simulink model "Esercizio7_sim"  (R2022a)
settings: Solver=VariableStepAuto  StartTime=0.0  StopTime=10  RelTol=1e-3
values from neighbouring files (symbols this model uses):
  C_d = c2d(C, Tc, 'tustin')    [Esercizio7.m]    (also in myESE6.m)
  G = tf(num, den)    [Esercizio7.m]    (also in myESE6.m = tf(num,den))
  Tc = 2*pi/ 500    (= 0.0125663706144)    [Esercizio7.m]    (also in SPIEGAZIONE.m = 2*PI/wc; myESE6.m)
settings Model: Creator=chiar  LastModifiedBy=Stefano
settings SolverCC: AlgebraicLoopSolver=TrustRegion
settings DebuggingCC: UnconnectedInputMsg=warning  UnconnectedOutputMsg=warning  UnconnectedLineMsg=warning  SFMachineParentedDataDiag=warning
settings RTWCC: DLArmComputeVersion=19.05

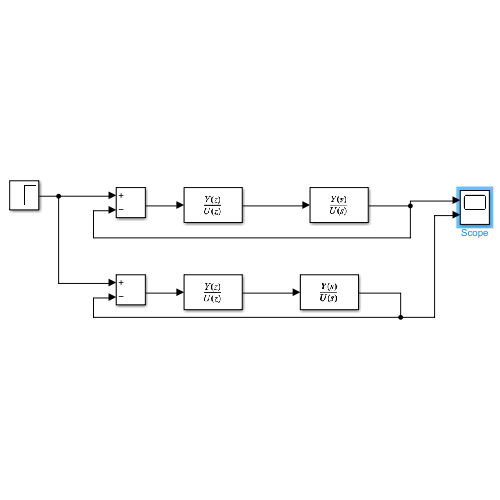
[thumbnail: Simulink's stored preview of the top-level diagram]
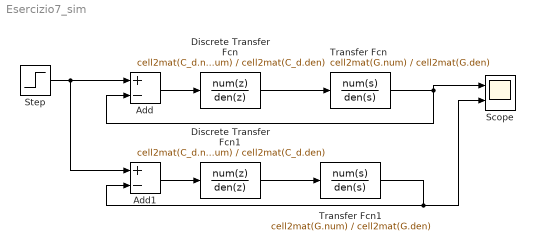
== system Esercizio7_sim ==
  Add : Sum  Inputs=+-
  Add1 : Sum  Inputs=+-
  Discrete Transfer Fcn : DiscreteTransferFcn  Numerator=cell2mat(C_d.num)  Denominator=cell2mat(C_d.den)  SampleTime=Tc
  Discrete Transfer Fcn1 : DiscreteTransferFcn  Numerator=cell2mat(C_d.num)  Denominator=cell2mat(C_d.den)  SampleTime=0.1
  Scope : Scope  NumInputPorts=2
  Step : Step  SampleTime=0
  Transfer Fcn : TransferFcn  Numerator=cell2mat(G.num)  Denominator=cell2mat(G.den)
  Transfer Fcn1 : TransferFcn  Numerator=cell2mat(G.num)  Denominator=cell2mat(G.den)
  wires:
  Discrete Transfer Fcn/1 -> Transfer Fcn/1
  Transfer Fcn/1 -> Add/2, Scope/1
  Add/1 -> Discrete Transfer Fcn/1
  Transfer Fcn1/1 -> Scope/2, Add1/2
  Add1/1 -> Discrete Transfer Fcn1/1
  Step/1 -> Add1/1, Add/1
  Discrete Transfer Fcn1/1 -> Transfer Fcn1/1
